simulink library "pump_and_fans_workingLibrary"  (R2020a)
settings: Solver=ode45  StartTime=0.0  StopTime=10.0  RelTol=1e-3  EnableMultiTasking=on
undefined symbols (not defined in the file): CR
libraries: simulink x2
settings Model: Creator=aldernl  LastModifiedBy=Harjot
settings DataIOCC: LimitDataPoints=on
settings OptimizationCC: LifeSpan=inf
settings DebuggingCC: AllowSymbolicDim=off  SFUnexpectedBacktrackingDiag=warning  SFNoUnconditionalDefaultTransitionDiag=warning  ArithmeticOperatorsInVariantConditions=warning
settings SFSimCC: SimUseLocalCustomCode=off  CustomCodeUndefinedFunction=UseInterfaceOnly
settings RTWCC: RTWUseLocalCustomCode=off
settings CodeAppCC: StateflowObjectComments=on
settings GRTTargetCC: TargetLangStandard=C89/C90 (ANSI)
settings ConfigComp: CovMetricSettings=dw  CovHtmlReporting=on  CovSaveCumulativeToWorkspaceVar=on  CovSaveSingleToWorkspaceVar=on  CovExternalEMLEnable=off

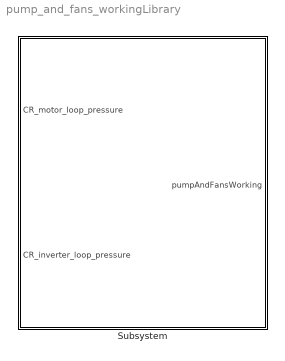
== system pump_and_fans_workingLibrary ==
  Subsystem : Subsystem

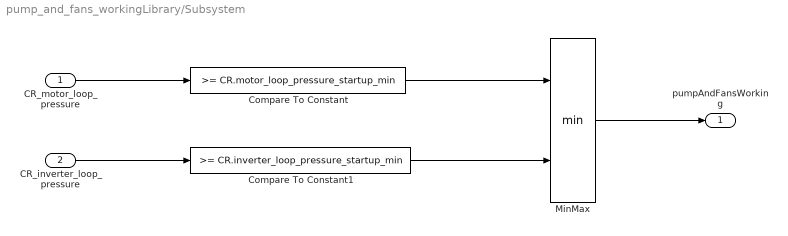
== system pump_and_fans_workingLibrary/Subsystem ==
  CR_motor_loop_pressure : Inport  OutDataTypeStr=double  PortDimensions=1
  CR_inverter_loop_pressure : Inport  Port=2  OutDataTypeStr=double  PortDimensions=1
  Compare To Constant : simulink/Logic and Bit Operations/Compare To Constant  relop=>=  const=CR.motor_loop_pressure_startup_min  OutDataTypeStr=uint8
  Compare To Constant1 : simulink/Logic and Bit Operations/Compare To Constant  relop=>=  const=CR.inverter_loop_pressure_startup_min  OutDataTypeStr=uint8
  MinMax : MinMax  Inputs=2  OutDataTypeStr=double
  pumpAndFansWorking : Outport  VectorParamsAs1DForOutWhenUnconnected=off
  wires:
  CR_motor_loop_pressure/1 -> Compare To Constant/1
  CR_inverter_loop_pressure/1 -> Compare To Constant1/1
  MinMax/1 -> pumpAndFansWorking/1
  Compare To Constant/1 -> MinMax/1
  Compare To Constant1/1 -> MinMax/2
